simulink model "W2P3"  (R2020b)
settings: Solver=ode45  StartTime=0.0  StopTime=120  RelTol=1e-3
undefined symbols (not defined in the file or in its folder): b, Kd, Ki, Kp, m
settings Model: Creator=ASUS  LastModifiedBy=ASUS

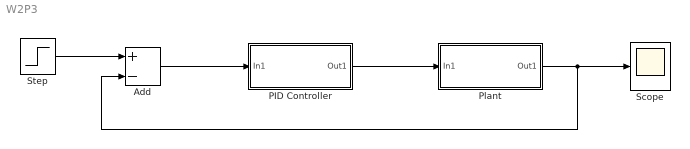
== system W2P3 ==
  Add : Sum  Inputs=+-
  PID Controller : Subsystem
  Plant : Subsystem
  Scope : Scope
  Step : Step  Time=0  After=500  SampleTime=0
  wires:
  Step/1 -> Add/1
  Plant/1(Out1) -> Add/2, Scope/1
  Add/1 -> PID Controller/1(In1)
  PID Controller/1(Out1) -> Plant/1(In1)

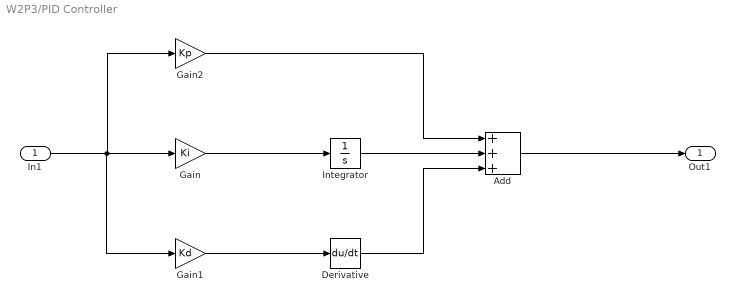
== system W2P3/PID Controller ==
  In1 : Inport
  Add : Sum  Inputs=+++
  Derivative : Derivative
  Gain : Gain  Gain=Ki
  Gain1 : Gain  Gain=Kd
  Gain2 : Gain  Gain=Kp
  Integrator : Integrator
  Out1 : Outport
  wires:
  In1/1 -> Gain1/1, Gain2/1, Gain/1
  Gain/1 -> Integrator/1
  Integrator/1 -> Add/2
  Gain2/1 -> Add/1
  Add/1 -> Out1/1
  Gain1/1 -> Derivative/1
  Derivative/1 -> Add/3

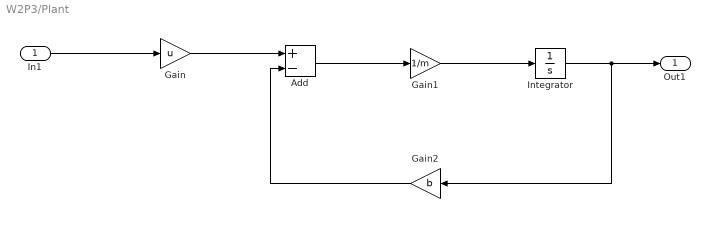
== system W2P3/Plant ==
  In1 : Inport
  Add : Sum  Inputs=+-
  Gain : Gain  Gain=u
  Gain1 : Gain  Gain=1/m
  Gain2 : Gain  Gain=b
  Integrator : Integrator
  Out1 : Outport
  wires:
  Gain/1 -> Add/1
  Add/1 -> Gain1/1
  In1/1 -> Gain/1
  Gain2/1 -> Add/2
  Gain1/1 -> Integrator/1
  Integrator/1 -> Gain2/1, Out1/1
